simulink model "testi_sim"  (R2020a)
settings: Solver=FixedStepAuto  StartTime=0.0  StopTime=25  FixedStep=0.001  RelTol=1e-3  EnableMultiTasking=on
values from neighbouring files (symbols this model uses):
  Jeq = Jm + Jh + Jd    (= 2.089856e-05)    [testi.m]
  km = 0.042    [testi.m]
  Kp = 1.2*10^(-27.5/20)    (= 0.0506035804114)    [testi.m]
  kt = 0.042    [testi.m]
  Rm = 8.4    [testi.m]
  Ti = 1/((km*kt)/(Rm*Jeq))    (= 0.099516952381)    [testi.m]
settings Model: Creator=pyrhonen  LastModifiedBy=lauri
settings DataIOCC: ReturnWorkspaceOutputs=off
settings OptimizationCC: LifeSpan=inf
settings DebuggingCC: SFUnexpectedBacktrackingDiag=warning  SFNoUnconditionalDefaultTransitionDiag=warning  ArithmeticOperatorsInVariantConditions=warning
settings SFSimCC: SimUseLocalCustomCode=off  CustomCodeUndefinedFunction=UseInterfaceOnly
settings RTWCC: RTWUseLocalCustomCode=off
settings CodeAppCC: StateflowObjectComments=on
settings GRTTargetCC: TargetLangStandard=C89/C90 (ANSI)
settings ConfigComp: CovMetricSettings=dw  CovHtmlReporting=on  CovSaveCumulativeToWorkspaceVar=on  CovSaveSingleToWorkspaceVar=on  CovExternalEMLEnable=off

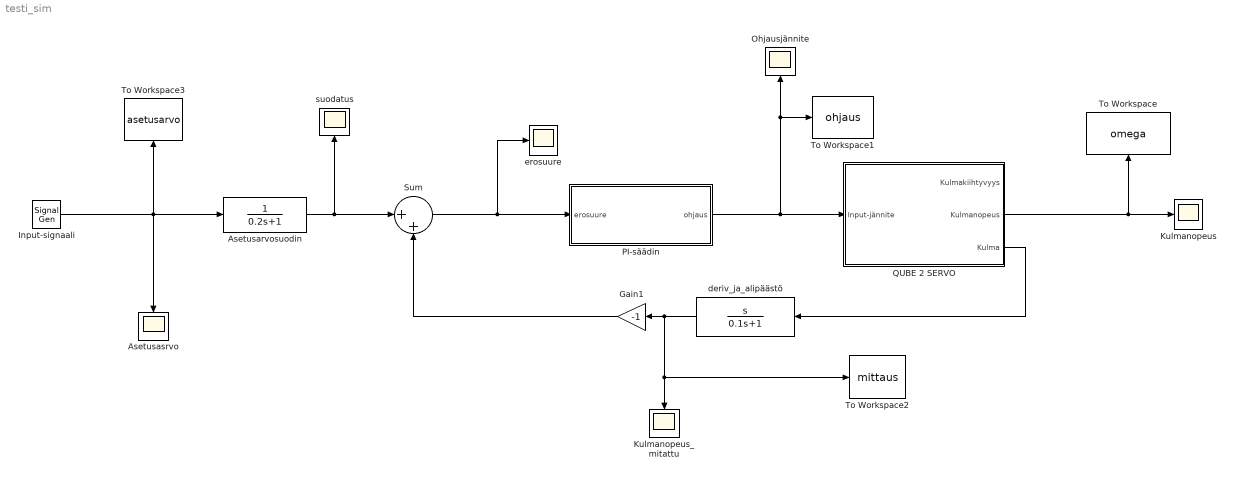
== system testi_sim ==
  Asetusarvosuodin : TransferFcn  Denominator=[0.2 1]
  Asetusasrvo : Scope
  Gain1 : Gain  Gain=-1
  Input-signaali : SignalGenerator  WaveForm=square  Amplitude=200  Frequency=0.4  Units=rad/sec
  Kulmanopeus : Scope
  Kulmanopeus_mitattu : Scope
  Ohjausjännite : Scope
  PI-säädin : Subsystem
  QUBE 2 SERVO : Subsystem
  Sum : Sum  Inputs=|++
  To Workspace : ToWorkspace  VariableName=omega  SaveFormat=Structure With Time  SampleTime=-1
  To Workspace1 : ToWorkspace  VariableName=ohjaus  SaveFormat=Structure With Time  SampleTime=-1
  To Workspace2 : ToWorkspace  VariableName=mittaus  SaveFormat=Structure With Time  SampleTime=-1
  To Workspace3 : ToWorkspace  VariableName=asetusarvo  SaveFormat=Structure With Time  SampleTime=-1
  deriv_ja_alipäästö : TransferFcn  Numerator=[1 0]  Denominator=[0.1 1]
  erosuure : Scope
  suodatus : Scope
  wires:
  QUBE 2 SERVO/2(Kulmanopeus) -> To Workspace/1, Kulmanopeus/1
  PI-säädin/1(ohjaus) -> QUBE 2 SERVO/1(Input-jännite), To Workspace1/1, Ohjausjännite/1
  Input-signaali/1 -> Asetusarvosuodin/1, Asetusasrvo/1, To Workspace3/1
  deriv_ja_alipäästö/1 -> Gain1/1, Kulmanopeus_mitattu/1, To Workspace2/1
  QUBE 2 SERVO/3(Kulma) -> deriv_ja_alipäästö/1
  Gain1/1 -> Sum/2
  Sum/1 -> erosuure/1, PI-säädin/1(erosuure)
  Asetusarvosuodin/1 -> suodatus/1, Sum/1

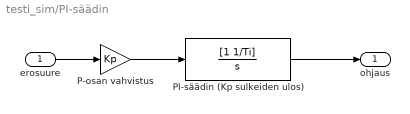
== system testi_sim/PI-säädin ==
  erosuure : Inport
  P-osan vahvistus : Gain  Gain=Kp
  PI-säädin (Kp sulkeiden ulos) : TransferFcn  Numerator=[1 1/Ti]  Denominator=[1 0]
  ohjaus : Outport
  wires:
  erosuure/1 -> P-osan vahvistus/1
  PI-säädin (Kp sulkeiden ulos)/1 -> ohjaus/1
  P-osan vahvistus/1 -> PI-säädin (Kp sulkeiden ulos)/1

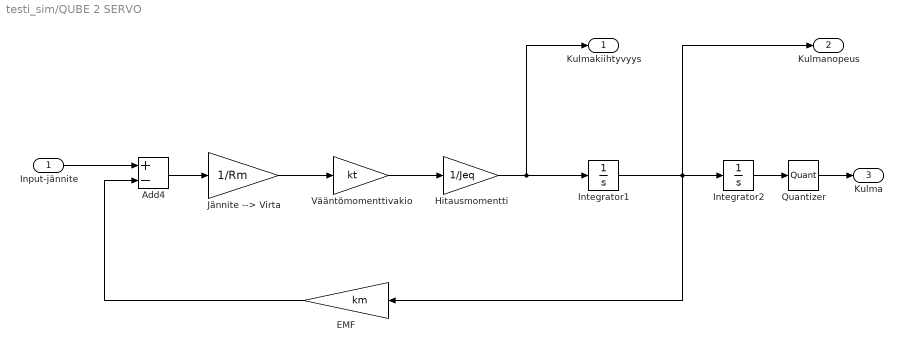
== system testi_sim/QUBE 2 SERVO ==
  Input-jännite : Inport
  Add4 : Sum  Inputs=+-
  EMF : Gain  Gain=km
  Hitausmomentti : Gain  Gain=1/Jeq
  Integrator1 : Integrator
  Integrator2 : Integrator
  Jännite --> Virta : Gain  Gain=1/Rm
  Quantizer : Quantizer  QuantizationInterval=1/512
  Vääntömomenttivakio : Gain  Gain=kt
  Kulmakiihtyvyys : Outport
  Kulmanopeus : Outport  Port=2
  Kulma : Outport  Port=3
  wires:
  Input-jännite/1 -> Add4/1
  Add4/1 -> Jännite --> Virta/1
  Jännite --> Virta/1 -> Vääntömomenttivakio/1
  EMF/1 -> Add4/2
  Integrator2/1 -> Quantizer/1
  Integrator1/1 -> Integrator2/1, EMF/1, Kulmanopeus/1
  Vääntömomenttivakio/1 -> Hitausmomentti/1
  Hitausmomentti/1 -> Kulmakiihtyvyys/1, Integrator1/1
  Quantizer/1 -> Kulma/1
